simulink library "CryoDetLibCMB"  (R2016b)
settings: Solver=VariableStepAuto  StartTime=0.0  StopTime=10.0  RelTol=1e-3
undefined symbols (not defined in the file): A, B, C, D, Fadc, Fclk, PCIN, xlipgetpartsetting
libraries: xbsIndex_r4 x640, CryoDetLibCMB x81, CryoDetLib x2, simulink x1
(part 11 of 12)

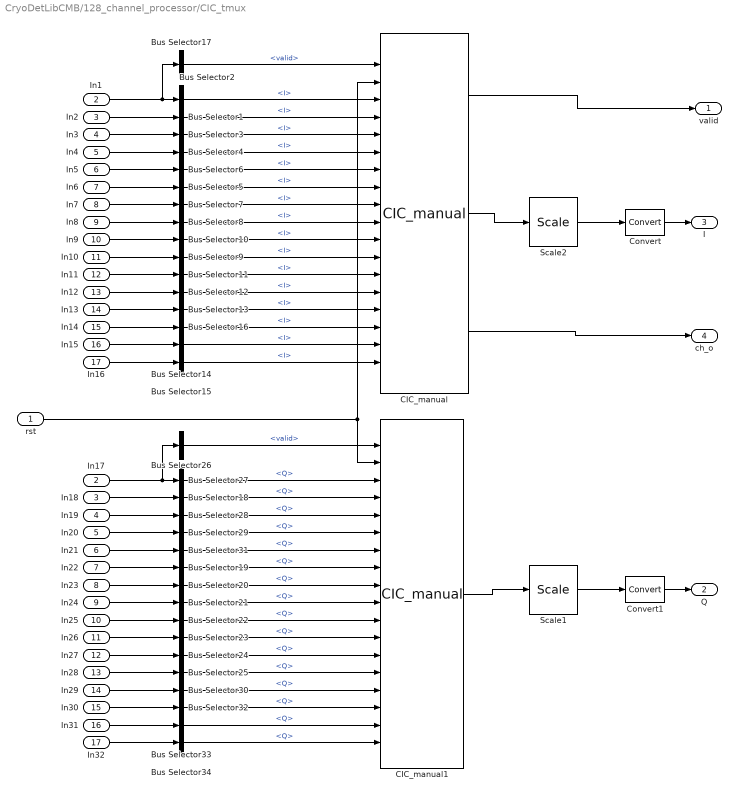
== system CryoDetLibCMB/128_channel_processor/CIC_tmux ==
  rst : Inport
  In1 : Inport  Port=2
  In2 : Inport  Port=3
  In3 : Inport  Port=4
  In4 : Inport  Port=5
  In5 : Inport  Port=6
  In6 : Inport  Port=7
  In7 : Inport  Port=8
  In8 : Inport  Port=9
  In9 : Inport  Port=10
  In10 : Inport  Port=11
  In11 : Inport  Port=12
  In12 : Inport  Port=13
  In13 : Inport  Port=14
  In14 : Inport  Port=15
  In15 : Inport  Port=16
  In16 : Inport  Port=17
  Bus Selector{1..16} (16 alike) : BusSelector  OutputSignals=I
  Bus Selector17 : BusSelector  OutputSignals=valid
  Bus Selector{18..25,27..34} (16 alike) : BusSelector  OutputSignals=Q
  Bus Selector26 : BusSelector  OutputSignals=valid
  CIC_manual : CryoDetLibCMB/CIC_manual  n_bit=30  b_pt=15
  CIC_manual1 : CryoDetLibCMB/CIC_manual  n_bit=30  b_pt=15
  Convert : xbsIndex_r4/Convert  gui_display_data_type=Fixed-point  arith_type="Signed  (2's comp)"  n_bits=18  bin_pt=16  float_type=Single  exp_bits=8  fraction_bits=24  quantization=Truncate  overflow=Wrap  en=off  latency=0  pipeline=off  dbl_ovrd=off  block_type=convert
  Convert1 : xbsIndex_r4/Convert  gui_display_data_type=Fixed-point  arith_type="Signed  (2's comp)"  n_bits=18  bin_pt=16  float_type=Single  exp_bits=8  fraction_bits=24  quantization=Truncate  overflow=Wrap  en=off  latency=0  pipeline=off  dbl_ovrd=off  block_type=convert
  In17 : InportShadow  Port=2
  In18 : InportShadow  Port=3
  In19 : InportShadow  Port=4
  In20 : InportShadow  Port=5
  In21 : InportShadow  Port=6
  In22 : InportShadow  Port=7
  In23 : InportShadow  Port=8
  In24 : InportShadow  Port=9
  In25 : InportShadow  Port=10
  In26 : InportShadow  Port=11
  In27 : InportShadow  Port=12
  In28 : InportShadow  Port=13
  In29 : InportShadow  Port=14
  In30 : InportShadow  Port=15
  In31 : InportShadow  Port=16
  In32 : InportShadow  Port=17
  Scale1 : xbsIndex_r4/Scale  scale_factor=-12  dbl_ovrd=off  block_type=scale
  Scale2 : xbsIndex_r4/Scale  scale_factor=-12  dbl_ovrd=off  block_type=scale
  valid : Outport
  Q : Outport  Port=2
  I : Outport  Port=3
  ch_o : Outport  Port=4
  wires:
  rst/1 -> CIC_manual1/2, CIC_manual/2
  Bus Selector26/1 -> CIC_manual1/1  "<valid>"
  Bus Selector34/1 -> CIC_manual1/18  "<Q>"
  Bus Selector33/1 -> CIC_manual1/17  "<Q>"
  Bus Selector32/1 -> CIC_manual1/16  "<Q>"
  Bus Selector31/1 -> CIC_manual1/7  "<Q>"
  Bus Selector30/1 -> CIC_manual1/15  "<Q>"
  Bus Selector29/1 -> CIC_manual1/6  "<Q>"
  Bus Selector28/1 -> CIC_manual1/5  "<Q>"
  Bus Selector27/1 -> CIC_manual1/3  "<Q>"
  Bus Selector25/1 -> CIC_manual1/14  "<Q>"
  Bus Selector24/1 -> CIC_manual1/13  "<Q>"
  Bus Selector23/1 -> CIC_manual1/12  "<Q>"
  Bus Selector22/1 -> CIC_manual1/11  "<Q>"
  Bus Selector21/1 -> CIC_manual1/10  "<Q>"
  Bus Selector20/1 -> CIC_manual1/9  "<Q>"
  Bus Selector19/1 -> CIC_manual1/8  "<Q>"
  Bus Selector18/1 -> CIC_manual1/4  "<Q>"
  In1/1 -> Bus Selector17/1, Bus Selector2/1
  In2/1 -> Bus Selector1/1
  In3/1 -> Bus Selector3/1
  In4/1 -> Bus Selector4/1
  In5/1 -> Bus Selector6/1
  In6/1 -> Bus Selector5/1
  In7/1 -> Bus Selector7/1
  In8/1 -> Bus Selector8/1
  In9/1 -> Bus Selector10/1
  In10/1 -> Bus Selector9/1
  In11/1 -> Bus Selector11/1
  In12/1 -> Bus Selector12/1
  In13/1 -> Bus Selector13/1
  In14/1 -> Bus Selector16/1
  In15/1 -> Bus Selector14/1
  In16/1 -> Bus Selector15/1
  In17/1 -> Bus Selector27/1, Bus Selector26/1
  In18/1 -> Bus Selector18/1
  In19/1 -> Bus Selector28/1
  In20/1 -> Bus Selector29/1
  In21/1 -> Bus Selector31/1
  In22/1 -> Bus Selector19/1
  In23/1 -> Bus Selector20/1
  In24/1 -> Bus Selector21/1
  In25/1 -> Bus Selector22/1
  In26/1 -> Bus Selector23/1
  In27/1 -> Bus Selector24/1
  In28/1 -> Bus Selector25/1
  In29/1 -> Bus Selector30/1
  In30/1 -> Bus Selector32/1
  In31/1 -> Bus Selector33/1
  In32/1 -> Bus Selector34/1
  Bus Selector1/1 -> CIC_manual/4  "<I>"
  Bus Selector10/1 -> CIC_manual/11  "<I>"
  Bus Selector11/1 -> CIC_manual/13  "<I>"
  Bus Selector12/1 -> CIC_manual/14  "<I>"
  Bus Selector13/1 -> CIC_manual/15  "<I>"
  Bus Selector14/1 -> CIC_manual/17  "<I>"
  Bus Selector15/1 -> CIC_manual/18  "<I>"
  Bus Selector16/1 -> CIC_manual/16  "<I>"
  Bus Selector17/1 -> CIC_manual/1  "<valid>"
  Bus Selector2/1 -> CIC_manual/3  "<I>"
  Bus Selector3/1 -> CIC_manual/5  "<I>"
  Bus Selector4/1 -> CIC_manual/6  "<I>"
  Bus Selector5/1 -> CIC_manual/8  "<I>"
  Bus Selector6/1 -> CIC_manual/7  "<I>"
  Bus Selector7/1 -> CIC_manual/9  "<I>"
  Bus Selector8/1 -> CIC_manual/10  "<I>"
  Bus Selector9/1 -> CIC_manual/12  "<I>"
  CIC_manual/2 -> Scale2/1
  CIC_manual/1 -> valid/1
  CIC_manual/3 -> ch_o/1
  CIC_manual1/2 -> Scale1/1
  Convert/1 -> I/1
  Convert1/1 -> Q/1
  Scale2/1 -> Convert/1
  Scale1/1 -> Convert1/1

== system CryoDetLibCMB/128_channel_processor/IQ_status_sel ==
  sel : Inport
  Q : Inport  Port=2
  I : Inport  Port=3
  ch : Inport  Port=4
  BitBasher : xbsIndex_r4/BitBasher  bitexpr=out = {I,Q}  display_expr=off  sr_1=out  arith_type1=Unsigned  bin_pt1=0  sr_2=2  arith_type2=Unsigned  bin_pt2=0  sr_3=3  arith_type3=Unsigned  bin_pt3=0  sr_4=4  arith_type4=Unsigned  bin_pt4=0  dbl_ovrd=off  block_type=bitbasher
  Convert : xbsIndex_r4/Convert  gui_display_data_type=Fixed-point  arith_type="Signed  (2's comp)"  n_bits=16  bin_pt=15  float_type=Single  exp_bits=8  fraction_bits=24  quantization=Truncate  overflow=Wrap  en=off  latency=1  pipeline=off  dbl_ovrd=off  block_type=convert
  Convert1 : xbsIndex_r4/Convert  gui_display_data_type=Fixed-point  arith_type="Signed  (2's comp)"  n_bits=16  bin_pt=15  float_type=Single  exp_bits=8  fraction_bits=24  quantization=Truncate  overflow=Wrap  en=off  latency=1  pipeline=off  dbl_ovrd=off  block_type=convert
  Register1 : xbsIndex_r4/Register  init=0  rst=off  en=on  dbl_ovrd=off  block_type=register
  Relational : xbsIndex_r4/Relational  mode=a=b  op_type=Bool  en=off  latency=1  dbl_ovrd=off  block_type=relational
  IQ_status_r : Outport
  wires:
  Convert/1 -> BitBasher/1
  sel/1 -> Relational/1
  ch/1 -> Relational/2
  Q/1 -> Convert/1
  I/1 -> Convert1/1
  BitBasher/1 -> Register1/1
  Register1/1 -> IQ_status_r/1
  Convert1/1 -> BitBasher/2
  Relational/1 -> Register1/2

== system CryoDetLibCMB/128_channel_processor/decimate_phase ==
  note: 1
  rst : Inport
  In1 : Inport  Port=2
  In2 : Inport  Port=3
  In3 : Inport  Port=4
  In4 : Inport  Port=5
  In5 : Inport  Port=6
  In6 : Inport  Port=7
  In7 : Inport  Port=8
  In8 : Inport  Port=9
  In9 : Inport  Port=10
  In10 : Inport  Port=11
  In11 : Inport  Port=12
  In12 : Inport  Port=13
  In13 : Inport  Port=14
  In14 : Inport  Port=15
  In15 : Inport  Port=16
  In16 : Inport  Port=17
  Bus Selector{1..16} (16 alike) : BusSelector  OutputSignals=phase
  Bus Selector17 : BusSelector  OutputSignals=valid
  decimate_128 : CryoDetLibCMB/decimate_128
  valid : Outport
  phase : Outport  Port=2
  ch_o : Outport  Port=3
  wires:
  rst/1 -> decimate_128/2
  In1/1 -> Bus Selector17/1, Bus Selector2/1
  In2/1 -> Bus Selector1/1
  In4/1 -> Bus Selector4/1
  In5/1 -> Bus Selector5/1
  In6/1 -> Bus Selector6/1
  In7/1 -> Bus Selector7/1
  In8/1 -> Bus Selector8/1
  In9/1 -> Bus Selector9/1
  In10/1 -> Bus Selector10/1
  In11/1 -> Bus Selector11/1
  In12/1 -> Bus Selector12/1
  In13/1 -> Bus Selector13/1
  In14/1 -> Bus Selector14/1
  In15/1 -> Bus Selector15/1
  In16/1 -> Bus Selector16/1
  Bus Selector1/1 -> decimate_128/4  "<phase>"
  Bus Selector9/1 -> decimate_128/11  "<phase>"
  Bus Selector11/1 -> decimate_128/13  "<phase>"
  Bus Selector12/1 -> decimate_128/14  "<phase>"
  Bus Selector13/1 -> decimate_128/15  "<phase>"
  Bus Selector15/1 -> decimate_128/17  "<phase>"
  Bus Selector16/1 -> decimate_128/18  "<phase>"
  Bus Selector14/1 -> decimate_128/16  "<phase>"
  Bus Selector17/1 -> decimate_128/1  "<valid>"
  Bus Selector2/1 -> decimate_128/3  "<phase>"
  In3/1 -> Bus Selector3/1
  Bus Selector4/1 -> decimate_128/6  "<phase>"
  Bus Selector6/1 -> decimate_128/8  "<phase>"
  Bus Selector5/1 -> decimate_128/7  "<phase>"
  Bus Selector7/1 -> decimate_128/9  "<phase>"
  Bus Selector8/1 -> decimate_128/10  "<phase>"
  Bus Selector10/1 -> decimate_128/12  "<phase>"
  decimate_128/2 -> phase/1
  Bus Selector3/1 -> decimate_128/5  "<phase>"
  decimate_128/1 -> valid/1
  decimate_128/3 -> ch_o/1

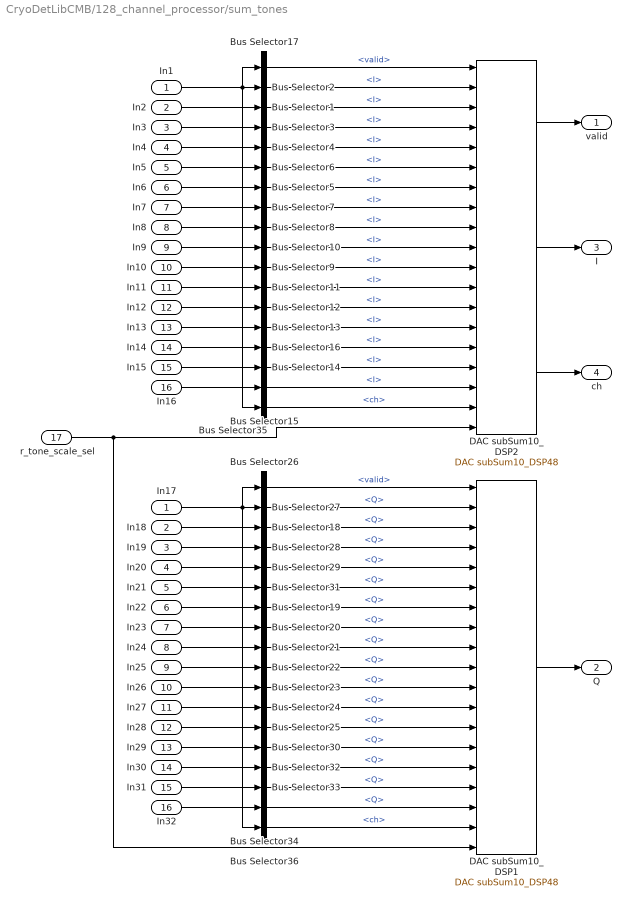
== system CryoDetLibCMB/128_channel_processor/sum_tones ==
  In1 : Inport
  In2 : Inport  Port=2
  In3 : Inport  Port=3
  In4 : Inport  Port=4
  In5 : Inport  Port=5
  In6 : Inport  Port=6
  In7 : Inport  Port=7
  In8 : Inport  Port=8
  In9 : Inport  Port=9
  In10 : Inport  Port=10
  In11 : Inport  Port=11
  In12 : Inport  Port=12
  In13 : Inport  Port=13
  In14 : Inport  Port=14
  In15 : Inport  Port=15
  In16 : Inport  Port=16
  r_tone_scale_sel : Inport  Port=17
  Bus Selector{1..16} (16 alike) : BusSelector  OutputSignals=I
  Bus Selector17 : BusSelector  OutputSignals=valid
  Bus Selector{18..25,27..34} (16 alike) : BusSelector  OutputSignals=Q
  Bus Selector26 : BusSelector  OutputSignals=valid
  Bus Selector35 : BusSelector  OutputSignals=ch
  Bus Selector36 : BusSelector  OutputSignals=ch
  DAC subSum10_DSP1 : CryoDetLibCMB/DAC subSum10_DSP48  VariantControl=Variant1
      link override Convert1: gui_display_data_type=Fixed-point  arith_type="Signed  (2's comp)"  n_bits=18  bin_pt=17  float_type=Single  exp_bits=8  fraction_bits=24  quantization=Truncate  overflow=Wrap  en=off  latency=0  pipeline=off  dbl_ovrd=off
      link override Convert2: gui_display_data_type=Fixed-point  arith_type="Signed  (2's comp)"  n_bits=19  bin_pt=17  float_type=Single  exp_bits=8  fraction_bits=24  quantization=Truncate  overflow=Wrap  en=off  latency=0  pipeline=off  dbl_ovrd=off
      link override Convert3: gui_display_data_type=Fixed-point  arith_type="Signed  (2's comp)"  n_bits=19  bin_pt=17  float_type=Single  exp_bits=8  fraction_bits=24  quantization=Truncate  overflow=Wrap  en=off  latency=0  pipeline=off  dbl_ovrd=off
      link override Convert4: gui_display_data_type=Fixed-point  arith_type="Signed  (2's comp)"  n_bits=18  bin_pt=17  float_type=Single  exp_bits=8  fraction_bits=24  quantization=Truncate  overflow=Wrap  en=off  latency=0  pipeline=off  dbl_ovrd=off
      link override Convert5: gui_display_data_type=Fixed-point  arith_type="Signed  (2's comp)"  n_bits=19  bin_pt=17  float_type=Single  exp_bits=8  fraction_bits=24  quantization=Truncate  overflow=Wrap  en=off  latency=0  pipeline=off  dbl_ovrd=off
      link override Convert6: gui_display_data_type=Fixed-point  arith_type="Signed  (2's comp)"  n_bits=19  bin_pt=17  float_type=Single  exp_bits=8  fraction_bits=24  quantization=Truncate  overflow=Wrap  en=off  latency=0  pipeline=off  dbl_ovrd=off
      link override Convert1: infoedit=Hardware notes: rounding and saturating require hardware resources; truncating and wrapping do not.
      link override Convert2: infoedit=Hardware notes: rounding and saturating require hardware resources; truncating and wrapping do not.
      link override Convert3: infoedit=Hardware notes: rounding and saturating require hardware resources; truncating and wrapping do not.
      link override Convert4: infoedit=Hardware notes: rounding and saturating require hardware resources; truncating and wrapping do not.
      link override Convert5: infoedit=Hardware notes: rounding and saturating require hardware resources; truncating and wrapping do not.
      link override Convert6: infoedit=Hardware notes: rounding and saturating require hardware resources; truncating and wrapping do not.
  DAC subSum10_DSP2 : CryoDetLibCMB/DAC subSum10_DSP48  VariantControl=Variant1
      link override Convert1: gui_display_data_type=Fixed-point  arith_type="Signed  (2's comp)"  n_bits=18  bin_pt=17  float_type=Single  exp_bits=8  fraction_bits=24  quantization=Truncate  overflow=Wrap  en=off  latency=0  pipeline=off  dbl_ovrd=off
      link override Convert2: gui_display_data_type=Fixed-point  arith_type="Signed  (2's comp)"  n_bits=19  bin_pt=17  float_type=Single  exp_bits=8  fraction_bits=24  quantization=Truncate  overflow=Wrap  en=off  latency=0  pipeline=off  dbl_ovrd=off
      link override Convert3: gui_display_data_type=Fixed-point  arith_type="Signed  (2's comp)"  n_bits=19  bin_pt=17  float_type=Single  exp_bits=8  fraction_bits=24  quantization=Truncate  overflow=Wrap  en=off  latency=0  pipeline=off  dbl_ovrd=off
      link override Convert4: gui_display_data_type=Fixed-point  arith_type="Signed  (2's comp)"  n_bits=18  bin_pt=17  float_type=Single  exp_bits=8  fraction_bits=24  quantization=Truncate  overflow=Wrap  en=off  latency=0  pipeline=off  dbl_ovrd=off
      link override Convert5: gui_display_data_type=Fixed-point  arith_type="Signed  (2's comp)"  n_bits=19  bin_pt=17  float_type=Single  exp_bits=8  fraction_bits=24  quantization=Truncate  overflow=Wrap  en=off  latency=0  pipeline=off  dbl_ovrd=off
      link override Convert6: gui_display_data_type=Fixed-point  arith_type="Signed  (2's comp)"  n_bits=19  bin_pt=17  float_type=Single  exp_bits=8  fraction_bits=24  quantization=Truncate  overflow=Wrap  en=off  latency=0  pipeline=off  dbl_ovrd=off
      link override Convert1: infoedit=Hardware notes: rounding and saturating require hardware resources; truncating and wrapping do not.
      link override Convert2: infoedit=Hardware notes: rounding and saturating require hardware resources; truncating and wrapping do not.
      link override Convert3: infoedit=Hardware notes: rounding and saturating require hardware resources; truncating and wrapping do not.
      link override Convert4: infoedit=Hardware notes: rounding and saturating require hardware resources; truncating and wrapping do not.
      link override Convert5: infoedit=Hardware notes: rounding and saturating require hardware resources; truncating and wrapping do not.
      link override Convert6: infoedit=Hardware notes: rounding and saturating require hardware resources; truncating and wrapping do not.
  In17 : InportShadow
  In18 : InportShadow  Port=2
  In19 : InportShadow  Port=3
  In20 : InportShadow  Port=4
  In21 : InportShadow  Port=5
  In22 : InportShadow  Port=6
  In23 : InportShadow  Port=7
  In24 : InportShadow  Port=8
  In25 : InportShadow  Port=9
  In26 : InportShadow  Port=10
  In27 : InportShadow  Port=11
  In28 : InportShadow  Port=12
  In29 : InportShadow  Port=13
  In30 : InportShadow  Port=14
  In31 : InportShadow  Port=15
  In32 : InportShadow  Port=16
  valid : Outport
  Q : Outport  Port=2
  I : Outport  Port=3
  ch : Outport  Port=4
  wires:
  In32/1 -> Bus Selector34/1
  In31/1 -> Bus Selector33/1
  In30/1 -> Bus Selector32/1
  In29/1 -> Bus Selector30/1
  In28/1 -> Bus Selector25/1
  In27/1 -> Bus Selector24/1
  In26/1 -> Bus Selector23/1
  In25/1 -> Bus Selector22/1
  In24/1 -> Bus Selector21/1
  In23/1 -> Bus Selector20/1
  In22/1 -> Bus Selector19/1
  In21/1 -> Bus Selector31/1
  In20/1 -> Bus Selector29/1
  In19/1 -> Bus Selector28/1
  In18/1 -> Bus Selector18/1
  In17/1 -> Bus Selector36/1, Bus Selector26/1, Bus Selector27/1
  In16/1 -> Bus Selector15/1
  In15/1 -> Bus Selector14/1
  In14/1 -> Bus Selector16/1
  In13/1 -> Bus Selector13/1
  In12/1 -> Bus Selector12/1
  In11/1 -> Bus Selector11/1
  In10/1 -> Bus Selector9/1
  In9/1 -> Bus Selector10/1
  In8/1 -> Bus Selector8/1
  In7/1 -> Bus Selector7/1
  In6/1 -> Bus Selector5/1
  In5/1 -> Bus Selector6/1
  In4/1 -> Bus Selector4/1
  In3/1 -> Bus Selector3/1
  In2/1 -> Bus Selector1/1
  In1/1 -> Bus Selector17/1, Bus Selector35/1, Bus Selector2/1
  Bus Selector35/1 -> DAC subSum10_DSP2/18  "<ch>"
  Bus Selector36/1 -> DAC subSum10_DSP1/18  "<ch>"
  DAC subSum10_DSP1/2 -> Q/1
  DAC subSum10_DSP2/3 -> ch/1
  DAC subSum10_DSP2/2 -> I/1
  DAC subSum10_DSP2/1 -> valid/1
  Bus Selector17/1 -> DAC subSum10_DSP2/1  "<valid>"
  Bus Selector7/1 -> DAC subSum10_DSP2/8  "<I>"
  Bus Selector1/1 -> DAC subSum10_DSP2/3  "<I>"
  Bus Selector16/1 -> DAC subSum10_DSP2/15  "<I>"
  Bus Selector12/1 -> DAC subSum10_DSP2/13  "<I>"
  Bus Selector14/1 -> DAC subSum10_DSP2/16  "<I>"
  Bus Selector8/1 -> DAC subSum10_DSP2/9  "<I>"
  Bus Selector4/1 -> DAC subSum10_DSP2/5  "<I>"
  Bus Selector11/1 -> DAC subSum10_DSP2/12  "<I>"
  Bus Selector3/1 -> DAC subSum10_DSP2/4  "<I>"
  Bus Selector6/1 -> DAC subSum10_DSP2/6  "<I>"
  Bus Selector15/1 -> DAC subSum10_DSP2/17  "<I>"
  Bus Selector13/1 -> DAC subSum10_DSP2/14  "<I>"
  Bus Selector2/1 -> DAC subSum10_DSP2/2  "<I>"
  Bus Selector10/1 -> DAC subSum10_DSP2/10  "<I>"
  Bus Selector5/1 -> DAC subSum10_DSP2/7  "<I>"
  Bus Selector9/1 -> DAC subSum10_DSP2/11  "<I>"
  Bus Selector20/1 -> DAC subSum10_DSP1/8  "<Q>"
  Bus Selector19/1 -> DAC subSum10_DSP1/7  "<Q>"
  Bus Selector28/1 -> DAC subSum10_DSP1/4  "<Q>"
  Bus Selector18/1 -> DAC subSum10_DSP1/3  "<Q>"
  Bus Selector21/1 -> DAC subSum10_DSP1/9  "<Q>"
  Bus Selector22/1 -> DAC subSum10_DSP1/10  "<Q>"
  Bus Selector23/1 -> DAC subSum10_DSP1/11  "<Q>"
  Bus Selector24/1 -> DAC subSum10_DSP1/12  "<Q>"
  Bus Selector25/1 -> DAC subSum10_DSP1/13  "<Q>"
  Bus Selector27/1 -> DAC subSum10_DSP1/2  "<Q>"
  Bus Selector31/1 -> DAC subSum10_DSP1/6  "<Q>"
  Bus Selector32/1 -> DAC subSum10_DSP1/15  "<Q>"
  Bus Selector33/1 -> DAC subSum10_DSP1/16  "<Q>"
  Bus Selector29/1 -> DAC subSum10_DSP1/5  "<Q>"
  Bus Selector34/1 -> DAC subSum10_DSP1/17  "<Q>"
  Bus Selector30/1 -> DAC subSum10_DSP1/14  "<Q>"
  Bus Selector26/1 -> DAC subSum10_DSP1/1  "<valid>"
  r_tone_scale_sel/1 -> DAC subSum10_DSP2/19, DAC subSum10_DSP1/19

== system CryoDetLibCMB/DDS Mixer/mixer ==
  note: depth 16 should be enough
      |   8 here
      |   ~3-4 in DDS block
  note: match latency for phaseBus
  note: Need complex? Swap IQ
  In1 : Inport
  In2 : Inport  Port=2
  phaseBus : Inport  Port=3
  BitBasher : xbsIndex_r4/BitBasher  bitexpr=out={ch, phase}  display_expr=off  sr_1=out  arith_type1=Unsigned  bin_pt1=0  sr_2=2  arith_type2=Unsigned  bin_pt2=0  sr_3=3  arith_type3=Unsigned  bin_pt3=0  sr_4=4  arith_type4=Unsigned  bin_pt4=0  dbl_ovrd=off  block_type=bitbasher
  BitBasher1 : xbsIndex_r4/BitBasher  bitexpr=|  display_expr=off  sr_1=ch  arith_type1=Unsigned  bin_pt1=0  sr_2=phase  arith_type2=Unsigned  bin_pt2=14  sr_3=3  arith_type3=Unsigned  bin_pt3=0  sr_4=4  arith_type4=Unsigned  bin_pt4=0  dbl_ovrd=off  block_type=bitbasher
      | ch = {in[2:0]}
      | phase = {in[16:3]}
  BitBasher2 : xbsIndex_r4/BitBasher  bitexpr=out={Q, I}  display_expr=off  sr_1=out  arith_type1=Unsigned  bin_pt1=0  sr_2=2  arith_type2=Unsigned  bin_pt2=0  sr_3=3  arith_type3=Unsigned  bin_pt3=0  sr_4=4  arith_type4=Unsigned  bin_pt4=0  dbl_ovrd=off  block_type=bitbasher
  BitBasher3 : xbsIndex_r4/BitBasher  bitexpr=|  display_expr=off  sr_1=Q  arith_type1="Signed  (2's comp)"  bin_pt1=15  sr_2=I  arith_type2="Signed  (2's comp)"  bin_pt2=15  sr_3=I  arith_type3=Unsigned  bin_pt3=0  sr_4=4  arith_type4=Unsigned  bin_pt4=0  dbl_ovrd=off  block_type=bitbasher
      | Q = {in[31:16]}
      | I = {in[15:0]}
  Bus Creator : BusCreator  Inputs=3
  Bus Creator1 : BusCreator  Inputs=4
  Bus Selector1 : BusSelector  OutputSignals=valid,Q,I,ch
  Bus Selector2 : BusSelector  OutputSignals=valid,Q,I
  Bus Selector3 : BusSelector  OutputSignals=valid,phase,ch
  "Complex Multiplier 6.0 " : xbsIndex_r4/Complex Multiplier 6.0   hasatlast=off  hasatuser=on  atuserwidth=3  hasbtlast=off  hasbtuser=off  btuserwidth=1  multtype=Use_Mults  optimizegoal=Resources  flowcontrol=NonBlocking  outputwidth=19  roundmode=Truncate  hasctrltlast=off  hasctrltuser=off  ctrltuserwidth=1  outtlastbehv=Null  latencyconfig=Manual  minimumlatency=6  aclken=off  aresetn=off  trim_axipin_name=on  simulation_type=hybrid_sim  simulation_model=sysgen:cmpy_v6_0  data_path_portlist={ 's_axis_a_tdata_real', 's_axis_a_tdata_imag', 's_axis_b_tdata_real', 's_axis_b_tdata_imag', 's_axis_ctrl_tdata_rounding_bit', 'm_axis_dout_tdata_real', 'm_axis_dout_tdata_imag' }  aportwidth=63  bportwidth=63  ip_name=Complex Multiplier  ip_version=6.0  dsptool_ready=true  ipcore_usecache=true  ipcore_useipmodelcache=true  ipcore_verbose=false  ipcore_latency_parameter='minimumlatency'  wrapper_available=true  port_translation_map={ 'aclken' => 'en', 'aresetn' => 'rst'}  block_type=cmpy_v6_0
  Convert : xbsIndex_r4/Convert  gui_display_data_type=Fixed-point  arith_type="Signed  (2's comp)"  n_bits=18  bin_pt=16  float_type=Single  exp_bits=8  fraction_bits=24  quantization=Truncate  overflow=Wrap  en=off  latency=0  pipeline=off  dbl_ovrd=off  block_type=convert
  Convert1 : xbsIndex_r4/Convert  gui_display_data_type=Fixed-point  arith_type="Signed  (2's comp)"  n_bits=18  bin_pt=16  float_type=Single  exp_bits=8  fraction_bits=24  quantization=Truncate  overflow=Wrap  en=off  latency=0  pipeline=off  dbl_ovrd=off  block_type=convert
  Delay : xbsIndex_r4/Delay  rst=off  infoeditControl=Selection of Reset will increase slice count due to use of real FFs and instead of SRLs  en=off  latency=14  reg_retiming=off  dbl_ovrd=off  block_type=delay
  Delay{1..4,8..11} (8 alike) : xbsIndex_r4/Delay  rst=off  infoeditControl=Selection of Reset will increase slice count due to use of real FFs and instead of SRLs  en=off  latency=1  reg_retiming=on  dbl_ovrd=off  block_type=delay
  Delay5 : xbsIndex_r4/Delay  rst=off  infoeditControl=Selection of Reset will increase slice count due to use of real FFs and instead of SRLs  en=off  latency=14  reg_retiming=off  dbl_ovrd=off  block_type=delay
  Delay6 : xbsIndex_r4/Delay  rst=off  infoeditControl=Selection of Reset will increase slice count due to use of real FFs and instead of SRLs  en=off  latency=15  reg_retiming=off  dbl_ovrd=off  block_type=delay
  Delay7 : xbsIndex_r4/Delay  rst=off  infoeditControl=Selection of Reset will increase slice count due to use of real FFs and instead of SRLs  en=off  latency=15  reg_retiming=off  dbl_ovrd=off  block_type=delay
  downmix : Outport
  phaseBus_o : Outport  Port=2
  wires:
  BitBasher/1 -> Delay7/1
  BitBasher2/1 -> Delay5/1
  BitBasher3/2 -> "Complex Multiplier 6.0 "/6
  Delay5/1 -> BitBasher3/1
  Bus Selector2/1 -> Delay/1  "<valid>"
  Bus Selector2/3 -> BitBasher2/2  "<I>"
  Bus Selector2/2 -> BitBasher2/1  "<Q>"
  Delay/1 -> "Complex Multiplier 6.0 "/5
  Delay2/1 -> "Complex Multiplier 6.0 "/1
  Bus Selector1/1 -> Delay2/1  "<valid>"
  In1/1 -> Bus Selector1/1
  Bus Selector1/2 -> Delay4/1  "<Q>"
  Delay4/1 -> "Complex Multiplier 6.0 "/2
  Bus Selector1/3 -> Delay3/1  "<I>"
  "Complex Multiplier 6.0 "/1 -> Delay8/1  "valid"
  "Complex Multiplier 6.0 "/4 -> Delay11/1  "INDX"
  Delay3/1 -> "Complex Multiplier 6.0 "/3
  "Complex Multiplier 6.0 "/2 -> Convert/1  "Q"
  Delay1/1 -> "Complex Multiplier 6.0 "/4
  BitBasher3/1 -> "Complex Multiplier 6.0 "/7
  "Complex Multiplier 6.0 "/3 -> Convert1/1  "I"
  In2/1 -> Bus Selector2/1
  Bus Selector1/4 -> Delay1/1  "<ch>"
  Convert/1 -> Delay9/1  "Q"
  Convert1/1 -> Delay10/1  "I"
  phaseBus/1 -> Bus Selector3/1
  Bus Selector3/1 -> Delay6/1  "<valid>"
  Bus Selector3/2 -> BitBasher/1  "<phase>"
  Bus Selector3/3 -> BitBasher/2  "<ch>"
  BitBasher1/1 -> Bus Creator/2  "ch"
  BitBasher1/2 -> Bus Creator/3  "phase"
  Delay7/1 -> BitBasher1/1
  Delay6/1 -> Bus Creator/1  "valid"
  Bus Creator/1 -> phaseBus_o/1
  Delay10/1 -> Bus Creator1/3  "I"
  Delay11/1 -> Bus Creator1/4  "ch"
  Delay8/1 -> Bus Creator1/1  "valid"
  Delay9/1 -> Bus Creator1/2  "Q"
  Bus Creator1/1 -> downmix/1

== system CryoDetLibCMB/DDS Mixer taylor series corrected/mixer ==
  note: depth 16 should be enough
      |   8 here
      |   ~3-4 in DDS block
  note: match latency for phaseBus
  note: Need complex? Swap IQ
  In1 : Inport
  In2 : Inport  Port=2
  phaseBus : Inport  Port=3
  BitBasher2 : xbsIndex_r4/BitBasher  bitexpr=out={Q, I}  display_expr=off  sr_1=out  arith_type1=Unsigned  bin_pt1=0  sr_2=2  arith_type2=Unsigned  bin_pt2=0  sr_3=3  arith_type3=Unsigned  bin_pt3=0  sr_4=4  arith_type4=Unsigned  bin_pt4=0  dbl_ovrd=off  block_type=bitbasher
  BitBasher3 : xbsIndex_r4/BitBasher  bitexpr=|  display_expr=off  sr_1=Q  arith_type1="Signed  (2's comp)"  bin_pt1=15  sr_2=I  arith_type2="Signed  (2's comp)"  bin_pt2=15  sr_3=I  arith_type3=Unsigned  bin_pt3=0  sr_4=4  arith_type4=Unsigned  bin_pt4=0  dbl_ovrd=off  block_type=bitbasher
      | Q = {in[31:16]}
      | I = {in[15:0]}
  Bus Creator : BusCreator  Inputs=3
  Bus Creator1 : BusCreator  Inputs=4
  Bus Selector1 : BusSelector  OutputSignals=valid,Q,I,ch
  Bus Selector2 : BusSelector  OutputSignals=valid,Q,I
  Bus Selector3 : BusSelector  OutputSignals=valid,phase,ch
  "Complex Multiplier 6.0 " : xbsIndex_r4/Complex Multiplier 6.0   hasatlast=off  hasatuser=on  atuserwidth=3  hasbtlast=off  hasbtuser=off  btuserwidth=1  multtype=Use_Mults  optimizegoal=Resources  flowcontrol=NonBlocking  outputwidth=19  roundmode=Truncate  hasctrltlast=off  hasctrltuser=off  ctrltuserwidth=1  outtlastbehv=Null  latencyconfig=Manual  minimumlatency=6  aclken=off  aresetn=off  trim_axipin_name=on  simulation_type=hybrid_sim  simulation_model=sysgen:cmpy_v6_0  data_path_portlist={ 's_axis_a_tdata_real', 's_axis_a_tdata_imag', 's_axis_b_tdata_real', 's_axis_b_tdata_imag', 's_axis_ctrl_tdata_rounding_bit', 'm_axis_dout_tdata_real', 'm_axis_dout_tdata_imag' }  aportwidth=63  bportwidth=63  ip_name=Complex Multiplier  ip_version=6.0  dsptool_ready=true  ipcore_usecache=true  ipcore_useipmodelcache=true  ipcore_verbose=false  ipcore_latency_parameter='minimumlatency'  wrapper_available=true  port_translation_map={ 'aclken' => 'en', 'aresetn' => 'rst'}  block_type=cmpy_v6_0
  Convert : xbsIndex_r4/Convert  gui_display_data_type=Fixed-point  arith_type="Signed  (2's comp)"  n_bits=18  bin_pt=16  float_type=Single  exp_bits=8  fraction_bits=24  quantization=Truncate  overflow=Wrap  en=off  latency=0  pipeline=off  dbl_ovrd=off  block_type=convert
  Convert1 : xbsIndex_r4/Convert  gui_display_data_type=Fixed-point  arith_type="Signed  (2's comp)"  n_bits=18  bin_pt=16  float_type=Single  exp_bits=8  fraction_bits=24  quantization=Truncate  overflow=Wrap  en=off  latency=0  pipeline=off  dbl_ovrd=off  block_type=convert
  Delay : xbsIndex_r4/Delay  rst=off  infoeditControl=Selection of Reset will increase slice count due to use of real FFs and instead of SRLs  en=off  latency=12  reg_retiming=off  dbl_ovrd=off  block_type=delay
  Delay{1..4,8..11} (8 alike) : xbsIndex_r4/Delay  rst=off  infoeditControl=Selection of Reset will increase slice count due to use of real FFs and instead of SRLs  en=off  latency=1  reg_retiming=on  dbl_ovrd=off  block_type=delay
  Delay12 : xbsIndex_r4/Delay  rst=off  infoeditControl=Selection of Reset will increase slice count due to use of real FFs and instead of SRLs  en=off  latency=16  reg_retiming=off  dbl_ovrd=off  block_type=delay
  Delay5 : xbsIndex_r4/Delay  rst=off  infoeditControl=Selection of Reset will increase slice count due to use of real FFs and instead of SRLs  en=off  latency=12  reg_retiming=off  dbl_ovrd=off  block_type=delay
  Delay6 : xbsIndex_r4/Delay  rst=off  infoeditControl=Selection of Reset will increase slice count due to use of real FFs and instead of SRLs  en=off  latency=16  reg_retiming=off  dbl_ovrd=off  block_type=delay
  Delay7 : xbsIndex_r4/Delay  rst=off  infoeditControl=Selection of Reset will increase slice count due to use of real FFs and instead of SRLs  en=off  latency=16  reg_retiming=off  dbl_ovrd=off  block_type=delay
  downmix : Outport
  phaseBus_o : Outport  Port=2
  wires:
  Delay12/1 -> Bus Creator/3  "ch"
  BitBasher2/1 -> Delay5/1
  BitBasher3/2 -> "Complex Multiplier 6.0 "/6
  Delay5/1 -> BitBasher3/1
  Bus Selector2/1 -> Delay/1  "<valid>"
  Bus Selector2/3 -> BitBasher2/2  "<I>"
  Bus Selector2/2 -> BitBasher2/1  "<Q>"
  Delay/1 -> "Complex Multiplier 6.0 "/5
  Delay2/1 -> "Complex Multiplier 6.0 "/1
  Bus Selector1/1 -> Delay2/1  "<valid>"
  In1/1 -> Bus Selector1/1
  Bus Selector1/2 -> Delay4/1  "<Q>"
  Delay4/1 -> "Complex Multiplier 6.0 "/2
  Bus Selector1/3 -> Delay3/1  "<I>"
  "Complex Multiplier 6.0 "/1 -> Delay8/1  "valid"
  "Complex Multiplier 6.0 "/4 -> Delay11/1  "INDX"
  Delay3/1 -> "Complex Multiplier 6.0 "/3
  "Complex Multiplier 6.0 "/2 -> Convert/1  "Q"
  Delay1/1 -> "Complex Multiplier 6.0 "/4
  BitBasher3/1 -> "Complex Multiplier 6.0 "/7
  "Complex Multiplier 6.0 "/3 -> Convert1/1  "I"
  In2/1 -> Bus Selector2/1
  Bus Selector1/4 -> Delay1/1  "<ch>"
  Convert/1 -> Delay9/1  "Q"
  Convert1/1 -> Delay10/1  "I"
  phaseBus/1 -> Bus Selector3/1
  Bus Selector3/1 -> Delay6/1  "<valid>"
  Bus Selector3/2 -> Delay7/1  "<phase>"
  Bus Selector3/3 -> Delay12/1  "<ch>"
  Delay7/1 -> Bus Creator/2  "phase"
  Delay6/1 -> Bus Creator/1  "valid"
  Bus Creator/1 -> phaseBus_o/1
  Delay10/1 -> Bus Creator1/3  "I"
  Delay11/1 -> Bus Creator1/4  "ch"
  Delay8/1 -> Bus Creator1/1  "valid"
  Delay9/1 -> Bus Creator1/2  "Q"
  Bus Creator1/1 -> downmix/1

== system CryoDetLibCMB/Loop Filter/initial Frequencies1 ==
  note: initial Frequencies
  note: select initial frequency
      | for now just mux from input registers
      | eventually configure RAM and loading protocol
  channel : Inport
  Gateway Out12 : xbsIndex_r4/Gateway Out  inherit_from_input=off  hdl_port=off  rows=1  columns=1  UseAsDAC=off  DACChannel='1'  interface=None  automatic_assignment=on  address_offset=hex2dec('00')  intf_name=''  intf_description=''  timing_constraint=None  locs_specified=off  LOCs={}  io_standard={}  block_type=gatewayout
  Gateway Out13 : xbsIndex_r4/Gateway Out  inherit_from_input=off  hdl_port=off  rows=1  columns=1  UseAsDAC=off  DACChannel='1'  interface=None  automatic_assignment=on  address_offset=hex2dec('00')  intf_name=''  intf_description=''  timing_constraint=None  locs_specified=off  LOCs={}  io_standard={}  block_type=gatewayout
  Mux : xbsIndex_r4/Mux  inputs=16  en=off  latency=1  precision=Full  arith_type=Unsigned  n_bits=24  bin_pt=24  quantization=Truncate  overflow=Wrap  dbl_ovrd=off  block_type=mux
  initial Freqs : Scope  NumInputPorts=2
  Fi : Outport
  wires:
  channel/1 -> Gateway Out12/1, Mux/1
  [F0] -> Mux/2
  [F1] -> Mux/3
  [F2] -> Mux/4
  [F3] -> Mux/5
  [F4] -> Mux/6
  [F5] -> Mux/7
  [F6] -> Mux/8
  [F7] -> Mux/9
  [F8] -> Mux/10
  [F9] -> Mux/11
  [F10] -> Mux/12
  [F11] -> Mux/13
  Mux/1 -> Gateway Out13/1, Fi/1
  Gateway Out13/1 -> initial Freqs/2
  Gateway Out12/1 -> initial Freqs/1
  [F15] -> Mux/17
  [F13] -> Mux/15
  [F12] -> Mux/14
  [F14] -> Mux/16

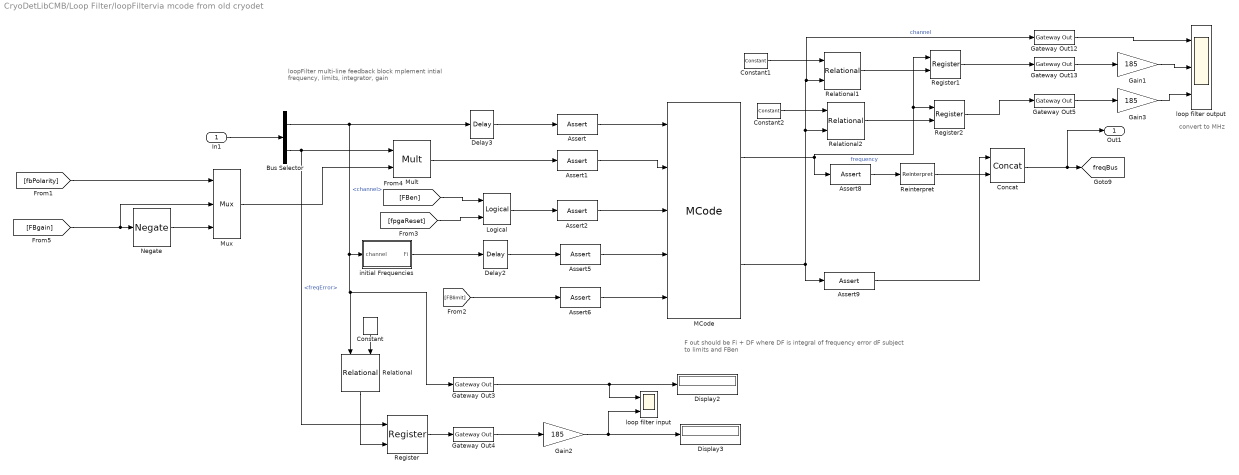
== system CryoDetLibCMB/Loop Filter/loopFiltervia mcode from old cryodet ==
  note: convert to MHz
  note: F out should be Fi + DF
      | where DF is integral of frequency error dF subject to limits and FBen
  note: loopFilter
      | multi-line feedback block
      | mplement intial frequency, limits, integrator, gain
  In1 : Inport
  Assert : xbsIndex_r4/Assert  assert_type=on  type_source=Explicitly  gui_display_data_type=Fixed-point  arith_type=Unsigned  n_bits=4  bin_pt=0  preci_type=Single  exp_width=8  frac_width=24  assert_rate=on  rate_source=Explicitly  period=Tclk  output_port=on  block_type=assert
  Assert1 : xbsIndex_r4/Assert  assert_type=on  type_source=Explicitly  gui_display_data_type=Fixed-point  arith_type="Signed  (2's comp)"  n_bits=32  bin_pt=30  preci_type=Single  exp_width=8  frac_width=24  assert_rate=on  rate_source=Explicitly  period=Tclk  output_port=on  block_type=assert
  Assert2 : xbsIndex_r4/Assert  assert_type=on  type_source=Explicitly  gui_display_data_type=Boolean  arith_type=Boolean  n_bits=16  bin_pt=14  preci_type=Single  exp_width=8  frac_width=24  assert_rate=on  rate_source=Explicitly  period=Tclk  output_port=on  block_type=assert
  Assert5 : xbsIndex_r4/Assert  assert_type=on  type_source=Explicitly  gui_display_data_type=Fixed-point  arith_type=Unsigned  n_bits=25  bin_pt=0  preci_type=Single  exp_width=8  frac_width=24  assert_rate=on  rate_source=Explicitly  period=Tclk  output_port=on  block_type=assert
  Assert6 : xbsIndex_r4/Assert  assert_type=on  type_source=Explicitly  gui_display_data_type=Fixed-point  arith_type=Unsigned  n_bits=16  bin_pt=16  preci_type=Single  exp_width=8  frac_width=24  assert_rate=on  rate_source=Explicitly  period=Tclk  output_port=on  block_type=assert
  Assert8 : xbsIndex_r4/Assert  assert_type=on  type_source=Explicitly  gui_display_data_type=Fixed-point  arith_type=Unsigned  n_bits=24  bin_pt=24  preci_type=Single  exp_width=8  frac_width=24  assert_rate=on  rate_source=Explicitly  period=Tclk  output_port=on  block_type=assert
  Assert9 : xbsIndex_r4/Assert  assert_type=on  type_source=Explicitly  gui_display_data_type=Fixed-point  arith_type=Unsigned  n_bits=4  bin_pt=0  preci_type=Single  exp_width=8  frac_width=24  assert_rate=on  rate_source=Explicitly  period=Tclk  output_port=on  block_type=assert
  Bus Selector : BusSelector  OutputSignals=channel,freqError
  Concat : xbsIndex_r4/Concat  num_inputs=2  dbl_ovrd=off  block_type=concat
  Constant : xbsIndex_r4/Constant  const=0  gui_display_data_type=Fixed-point  arith_type=Unsigned  n_bits=4  bin_pt=0  preci_type=Single  exp_width=8  frac_width=24  explicit_period=off  period=1  equ=P=C  opselect=C  inp2=PCIN>>17  opr=+  inp1=P  carry=CIN  dbl_ovrd=off  block_type=constant
  Constant1 : xbsIndex_r4/Constant  const=0  gui_display_data_type=Fixed-point  arith_type=Unsigned  n_bits=4  bin_pt=0  preci_type=Single  exp_width=8  frac_width=24  explicit_period=off  period=1  equ=P=C  opselect=C  inp2=PCIN>>17  opr=+  inp1=P  carry=CIN  dbl_ovrd=off  block_type=constant
  Constant2 : xbsIndex_r4/Constant  const=6  gui_display_data_type=Fixed-point  arith_type=Unsigned  n_bits=4  bin_pt=0  preci_type=Single  exp_width=8  frac_width=24  explicit_period=off  period=1  equ=P=C  opselect=C  inp2=PCIN>>17  opr=+  inp1=P  carry=CIN  dbl_ovrd=off  block_type=constant
  Delay2 : xbsIndex_r4/Delay  rst=off  infoeditControl=Selection of Reset will increase slice count due to use of real FFs and instead of SRLs  en=off  latency=3  reg_retiming=off  dbl_ovrd=off  block_type=delay
  Delay3 : xbsIndex_r4/Delay  rst=off  infoeditControl=Selection of Reset will increase slice count due to use of real FFs and instead of SRLs  en=off  latency=3  reg_retiming=off  dbl_ovrd=off  block_type=delay
  Display2 : Display
  Display3 : Display
  Gain1 : Gain  Gain=185
  Gain2 : Gain  Gain=185
  Gain3 : Gain  Gain=185
  Gateway Out12 : xbsIndex_r4/Gateway Out  inherit_from_input=off  hdl_port=off  rows=1  columns=1  UseAsDAC=off  DACChannel='1'  interface=None  automatic_assignment=on  address_offset=hex2dec('00')  intf_name=''  intf_description=''  timing_constraint=None  locs_specified=off  LOCs={}  io_standard={}  block_type=gatewayout
  Gateway Out13 : xbsIndex_r4/Gateway Out  inherit_from_input=on  hdl_port=off  rows=1  columns=1  UseAsDAC=off  DACChannel='1'  interface=None  automatic_assignment=on  address_offset=hex2dec('00')  intf_name=''  intf_description=''  timing_constraint=None  locs_specified=off  LOCs={}  io_standard={}  block_type=gatewayout
  Gateway Out3 : xbsIndex_r4/Gateway Out  inherit_from_input=off  hdl_port=off  rows=1  columns=1  UseAsDAC=off  DACChannel='1'  interface=None  automatic_assignment=on  address_offset=hex2dec('00')  intf_name=''  intf_description=''  timing_constraint=None  locs_specified=off  LOCs={}  io_standard={}  block_type=gatewayout
  Gateway Out4 : xbsIndex_r4/Gateway Out  inherit_from_input=off  hdl_port=off  rows=1  columns=1  UseAsDAC=off  DACChannel='1'  interface=None  automatic_assignment=on  address_offset=hex2dec('00')  intf_name=''  intf_description=''  timing_constraint=None  locs_specified=off  LOCs={}  io_standard={}  block_type=gatewayout
  Gateway Out5 : xbsIndex_r4/Gateway Out  inherit_from_input=on  hdl_port=off  rows=1  columns=1  UseAsDAC=off  DACChannel='1'  interface=None  automatic_assignment=on  address_offset=hex2dec('00')  intf_name=''  intf_description=''  timing_constraint=None  locs_specified=off  LOCs={}  io_standard={}  block_type=gatewayout
  Logical : xbsIndex_r4/Logical  logical_function=OR  inputs=2  en=off  latency=3  precision=User Defined  arith_type=Boolean  n_bits=16  bin_pt=0  align_bp=on  dbl_ovrd=off  block_type=logical
  MCode : xbsIndex_r4/MCode  mfname=multiLineFeedback  explicit_period=on  period=Tclk  inputsTable={'boundInpExpr'=>['','','','',''],'inputs'=>['channelNo','deltaF','FBen','Finitial','dFmax']}  outputsTable={'outputs'=>['freq','chanOut'],'suppressOut'=>['off','off']}  enable_stdout=off  enable_debug=off  suppress_output=on  defparams={}  hide_port_list={}  dbl_ovrd=off  block_type=mcode
  Mult : xbsIndex_r4/Mult  precision=User Defined  arith_type="Signed  (2's comp)"  n_bits=32  bin_pt=30  quantization=Truncate  overflow=Saturate  en=off  latency=3  use_behavioral_HDL=off  opt=Speed  use_embedded=on  optimum_pipeline=off  pipeline=on  dbl_ovrd=off  use_rpm=on  placement_style=Triangular  block_type=mult
  Mux : xbsIndex_r4/Mux  inputs=2  en=off  latency=1  precision=Full  arith_type=Unsigned  n_bits=16  bin_pt=14  quantization=Truncate  overflow=Wrap  dbl_ovrd=off  block_type=mux
  Negate : xbsIndex_r4/Negate  precision=Full  arith_type=Unsigned  n_bits=16  bin_pt=14  quantization=Truncate  overflow=Wrap  en=off  latency=1  dbl_ovrd=off  block_type=negate
  Register : xbsIndex_r4/Register  init=0  rst=off  en=on  dbl_ovrd=off  block_type=register
  Register1 : xbsIndex_r4/Register  init=0  rst=off  en=on  dbl_ovrd=off  block_type=register
  Register2 : xbsIndex_r4/Register  init=0  rst=off  en=on  dbl_ovrd=off  block_type=register
  Reinterpret : xbsIndex_r4/Reinterpret  force_arith_type=off  arith_type=Unsigned  force_bin_pt=on  bin_pt=0  block_type=reinterpret
  Relational : xbsIndex_r4/Relational  mode=a=b  op_type=Bool  en=off  latency=0  dbl_ovrd=off  block_type=relational
  Relational1 : xbsIndex_r4/Relational  mode=a=b  op_type=Bool  en=off  latency=0  dbl_ovrd=off  block_type=relational
  Relational2 : xbsIndex_r4/Relational  mode=a=b  op_type=Bool  en=off  latency=0  dbl_ovrd=off  block_type=relational
  initial Frequencies : Subsystem
  loop filter input : Scope  NumInputPorts=2
  loop filter output : Scope  NumInputPorts=3
  Out1 : Outport
  tag scope: freqBus=global
  wires:
  In1/1 -> Bus Selector/1
  Bus Selector/1 -> Relational/1, Gateway Out3/1, initial Frequencies/1(channel), Delay3/1  "<channel>"
  Bus Selector/2 -> Mult/1, Register/1  "<freqError>"
  MCode/2 -> Assert9/1, Relational2/2, Gateway Out12/1, Relational1/2  "channel"
  MCode/1 -> Assert8/1, Register2/1, Register1/1  "frequency"
  Concat/1 -> [freqBus], Out1/1
  [fbPolarity] -> Mux/1
  [FBgain] -> Mux/2, Negate/1
  [FBlimit] -> Assert6/1
  initial Frequencies/1(Fi) -> Delay2/1
  Assert/1 -> MCode/1
  Assert1/1 -> MCode/2
  Assert2/1 -> MCode/3
  Assert5/1 -> MCode/4
  Assert6/1 -> MCode/5
  Assert9/1 -> Concat/1
  Assert8/1 -> Reinterpret/1
  Reinterpret/1 -> Concat/2
  Gateway Out13/1 -> Gain1/1
  Gateway Out12/1 -> loop filter output/1
  Gateway Out4/1 -> Gain2/1
  Gateway Out3/1 -> loop filter input/1, Display2/1
  Constant/1 -> Relational/2
  Relational/1 -> Register/2
  Register/1 -> Gateway Out4/1
  Constant1/1 -> Relational1/1
  Relational1/1 -> Register1/2
  Register1/1 -> Gateway Out13/1
  Gain1/1 -> loop filter output/2
  Gain2/1 -> Display3/1, loop filter input/2
  Constant2/1 -> Relational2/1
  Relational2/1 -> Register2/2
  Register2/1 -> Gateway Out5/1
  Gateway Out5/1 -> Gain3/1
  Gain3/1 -> loop filter output/3
  Negate/1 -> Mux/3
  Mult/1 -> Assert1/1
  Mux/1 -> Mult/2
  [fpgaReset] -> Logical/2
  [FBen] -> Logical/1
  Logical/1 -> Assert2/1
  Delay3/1 -> Assert/1
  Delay2/1 -> Assert5/1

== system CryoDetLibCMB/dF/eta Mux ==
  note: eta Mux
  note: get calibration const for this channel
      | for now just mux from input registers
      | eventually configure RAM and loading protocol
  channel : Inport
  Bus Creator : BusCreator  Inputs=2
  Gateway Out1 : xbsIndex_r4/Gateway Out  inherit_from_input=off  hdl_port=off  rows=1  columns=1  UseAsDAC=off  DACChannel='1'  interface=None  automatic_assignment=on  address_offset=hex2dec('00')  intf_name=''  intf_description=''  timing_constraint=None  locs_specified=off  LOCs={}  io_standard={}  block_type=gatewayout
  Gateway Out12 : xbsIndex_r4/Gateway Out  inherit_from_input=off  hdl_port=off  rows=1  columns=1  UseAsDAC=off  DACChannel='1'  interface=None  automatic_assignment=on  address_offset=hex2dec('00')  intf_name=''  intf_description=''  timing_constraint=None  locs_specified=off  LOCs={}  io_standard={}  block_type=gatewayout
  Gateway Out13 : xbsIndex_r4/Gateway Out  inherit_from_input=off  hdl_port=off  rows=1  columns=1  UseAsDAC=off  DACChannel='1'  interface=None  automatic_assignment=on  address_offset=hex2dec('00')  intf_name=''  intf_description=''  timing_constraint=None  locs_specified=off  LOCs={}  io_standard={}  block_type=gatewayout
  Mux : xbsIndex_r4/Mux  inputs=16  en=off  latency=1  precision=Full  arith_type=Unsigned  n_bits=24  bin_pt=24  quantization=Truncate  overflow=Wrap  dbl_ovrd=off  block_type=mux
  Mux1 : xbsIndex_r4/Mux  inputs=16  en=off  latency=1  precision=Full  arith_type=Unsigned  n_bits=24  bin_pt=24  quantization=Truncate  overflow=Wrap  dbl_ovrd=off  block_type=mux
  eta scope : Scope  NumInputPorts=3
  eta out : Outport
  wires:
  channel/1 -> Mux/1, Gateway Out12/1, Mux1/1
  [reEta0] -> Mux/2
  [reEta1] -> Mux/3
  [reEta2] -> Mux/4
  [reEta3] -> Mux/5
  [reEta4] -> Mux/6
  [reEta5] -> Mux/7
  [reEta6] -> Mux/8
  [reEta7] -> Mux/9
  [reEta8] -> Mux/10
  [reEta9] -> Mux/11
  [reEta10] -> Mux/12
  [reEta11] -> Mux/13
  Mux/1 -> Bus Creator/1, Gateway Out13/1  "etaMag"
  Gateway Out13/1 -> eta scope/2
  Gateway Out12/1 -> eta scope/1
  [imEta0] -> Mux1/2
  [imEta1] -> Mux1/3
  [imEta2] -> Mux1/4
  [imEta3] -> Mux1/5
  [imEta4] -> Mux1/6
  [imEta5] -> Mux1/7
  [imEta6] -> Mux1/8
  [imEta7] -> Mux1/9
  [imEta8] -> Mux1/10
  [imEta9] -> Mux1/11
  [imEta10] -> Mux1/12
  [imEta11] -> Mux1/13
  Mux1/1 -> Bus Creator/2, Gateway Out1/1  "etaPhase"
  Gateway Out1/1 -> eta scope/3
  Bus Creator/1 -> eta out/1
  [reEta15] -> Mux/17
  [reEta14] -> Mux/16
  [reEta13] -> Mux/15
  [reEta12] -> Mux/14
  [imEta12] -> Mux1/14
  [imEta13] -> Mux1/15
  [imEta14] -> Mux1/16
  [imEta15] -> Mux1/17

== system CryoDetLibCMB/dF/ref phase RAM ==
  ref Phase : Inport
  read channel : Inport  Port=2
  Bus Creator1 : BusCreator  Inputs=2
  Bus Selector5 : BusSelector  OutputSignals=channel,refPhase
  Delay1 : xbsIndex_r4/Delay  rst=off  infoeditControl=Selection of Reset will increase slice count due to use of real FFs and instead of SRLs  en=off  latency=1  reg_retiming=off  dbl_ovrd=off  block_type=delay
  Dual Port RAM : xbsIndex_r4/Dual Port RAM  depth=16  initVector=0  distributed_mem=Distributed memory  init_a=0  init_b=0  rst_a=off  rst_b=off  en_a=off  en_b=off  latency=1  write_mode_A=Read Before Write  write_mode_B=Read After Write  optimize=Area  dbl_ovrd=off  block_type=dpram
  Terminator : Terminator
  write : xbsIndex_r4/Constant  const=1.0  gui_display_data_type=Boolean  arith_type=Boolean  n_bits=16  bin_pt=14  preci_type=Single  exp_width=8  frac_width=24  explicit_period=off  period=1  equ=P=C  opselect=C  inp2=PCIN>>17  opr=+  inp1=P  carry=CIN  dbl_ovrd=off  block_type=constant
  ref phase : Outport
  wires:
  write/1 -> Dual Port RAM/3
  Delay1/1 -> Bus Creator1/1  "chan"
  Dual Port RAM/2 -> Bus Creator1/2  "ref phase"
  Bus Creator1/1 -> ref phase/1
  read channel/1 -> Dual Port RAM/4, Delay1/1
  Dual Port RAM/1 -> Terminator/1
  ref Phase/1 -> Bus Selector5/1
  Bus Selector5/1 -> Dual Port RAM/1  "<channel>"
  Bus Selector5/2 -> Dual Port RAM/2  "<refPhase>"

== system CryoDetLibCMB/dF/ref phase diff ==
  note: ref phase diff
      | calulates difference in phase between present phase of DDS generating tone for a resonator and its phase when the signal now being recieved was generated.
      | That is this pahse difference is the integral of the frequency history of the tone generaotr over the ADC/DAC/cable/cryo latency
  note: ref delay is ADC/DAC/cryo latency in units of Fclk/16
  ref phase : Inport
  AddSub : xbsIndex_r4/AddSub  mode=Subtraction  use_carryin=off  use_carryout=off  en=off  latency=1  precision=Full  arith_type=Unsigned  n_bits=16  bin_pt=14  quantization=Truncate  overflow=Wrap  use_behavioral_HDL=off  hw_selection=Fabric  pipelined=off  dbl_ovrd=off  block_type=addsub
  Addressable Shift Register : xbsIndex_r4/Addressable Shift Register  infer_latency=on  depth=2  initVector=[0]  en=off  use_behavioral_HDL=off  Optimization=Resource  dbl_ovrd=off  block_type=addrsr
      settings: infoedit="Delay of configurable length.  Any element in the delay line can be addressed and driven onto the output port.<br><br>Hardware notes: Generates fast, compact FIFO-style shift registers or delay lines using SRL16/SRL32 mode of the slice LUTs"
  Bus Creator2 : BusCreator  Inputs=2
  Bus Selector5 : BusSelector  OutputSignals=channel,DDS Ref
  Delay : xbsIndex_r4/Delay  rst=off  infoeditControl=Selection of Reset will increase slice count due to use of real FFs and instead of SRLs  en=off  latency=1  reg_retiming=off  dbl_ovrd=off  block_type=delay
  Delay2 : xbsIndex_r4/Delay  rst=off  infoeditControl=Selection of Reset will increase slice count due to use of real FFs and instead of SRLs  en=off  latency=1  reg_retiming=off  dbl_ovrd=off  block_type=delay
  Shift : xbsIndex_r4/Shift  shift_dir=Left  shift_bits=4  en=off  latency=0  precision=User Defined  arith_type=Unsigned  n_bits=8  bin_pt=0  quantization=Truncate  overflow=Wrap  dbl_ovrd=off  block_type=shift
  phase diff : Outport
  wires:
  ref phase/1 -> Bus Selector5/1
  [refDel] -> Shift/1
  Shift/1 -> Addressable Shift Register/2
  Addressable Shift Register/1 -> AddSub/2
  Bus Selector5/2 -> AddSub/1, Addressable Shift Register/1  "<DDS Ref>"
  Delay/1 -> Delay2/1
  Bus Selector5/1 -> Delay/1  "<channel>"
  Delay2/1 -> Bus Creator2/1  "channel"
  AddSub/1 -> Bus Creator2/2  "refPhase"
  Bus Creator2/1 -> phase diff/1

== system CryoDetLibCMB/dF1/Subsystem ==
  note: default I/Q swap negates sense of rotation
  sel : Inport
  Q : Inport  Port=2
  I : Inport  Port=3
  Mux : xbsIndex_r4/Mux  inputs=2  en=off  latency=1  precision=Full  arith_type=Unsigned  n_bits=16  bin_pt=14  quantization=Truncate  overflow=Wrap  dbl_ovrd=off  block_type=mux
  Mux1 : xbsIndex_r4/Mux  inputs=2  en=off  latency=1  precision=Full  arith_type=Unsigned  n_bits=16  bin_pt=14  quantization=Truncate  overflow=Wrap  dbl_ovrd=off  block_type=mux
  Out1 : Outport
  Out2 : Outport  Port=2
  wires:
  sel/1 -> Mux1/1, Mux/1
  Mux/1 -> Out1/1
  Mux1/1 -> Out2/1
  I/1 -> Mux1/3, Mux/2
  Q/1 -> Mux/3, Mux1/2

== system CryoDetLibCMB/decimate_128/Subsystem ==
  sel : Inport
  sync : Inport  Port=2
  in : Inport  Port=3
  Mux1 : xbsIndex_r4/Mux  inputs=8  en=off  latency=1  precision=Full  arith_type=Unsigned  n_bits=16  bin_pt=14  quantization=Truncate  overflow=Wrap  dbl_ovrd=off  block_type=mux
  Register{,1..7} (8 alike) : xbsIndex_r4/Register  init=0  rst=off  en=on  dbl_ovrd=off  block_type=register
  Register{8..14} (7 alike) : xbsIndex_r4/Register  init=0  rst=off  en=off  dbl_ovrd=off  block_type=register
  o : Outport
  wires:
  Register11/1 -> Register4/2, Register12/1
  Mux1/1 -> o/1
  Register14/1 -> Register7/2
  Register1/1 -> Mux1/3
  Register2/1 -> Mux1/4
  in/1 -> Register/1, Register7/1, Register6/1, Register5/1, Register4/1, Register3/1, Register2/1, Register1/1
  Register13/1 -> Register6/2, Register14/1
  sync/1 -> Register/2, Register8/1
  Register6/1 -> Mux1/8
  Register4/1 -> Mux1/6
  Register8/1 -> Register1/2, Register9/1
  Register12/1 -> Register5/2, Register13/1
  Register3/1 -> Mux1/5
  Register7/1 -> Mux1/9
  Register/1 -> Mux1/2
  Register10/1 -> Register3/2, Register11/1
  sel/1 -> Mux1/1
  Register5/1 -> Mux1/7
  Register9/1 -> Register2/2, Register10/1
